simulink model "untitled"  (R2021a)
settings: Solver=VariableStepAuto  StartTime=0.0  StopTime=10.0  RelTol=1e-3
settings Model: Creator=ThinkPad  LastModifiedBy=ThinkPad

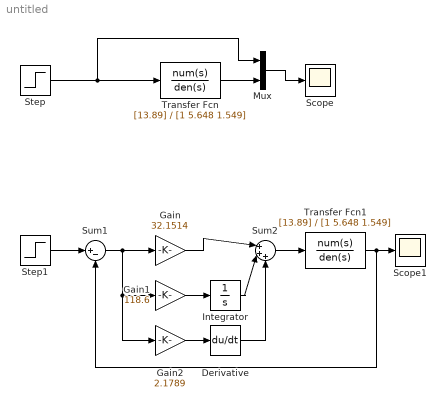
== system untitled ==
  Derivative : Derivative
  Gain : Gain  Gain=32.1514
  Gain1 : Gain  Gain=118.6
  Gain2 : Gain  Gain=2.1789
  Integrator : Integrator
  Mux : Mux  Inputs=2
  Scope : Scope
  Scope1 : Scope
  Step : Step  SampleTime=0
  Step1 : Step  SampleTime=0
  Sum1 : Sum  Inputs=|+-
  Sum2 : Sum  Inputs=|+++
  Transfer Fcn : TransferFcn  Numerator=[13.89]  Denominator=[1 5.648 1.549]
  Transfer Fcn1 : TransferFcn  Numerator=[13.89]  Denominator=[1 5.648 1.549]
  wires:
  Step/1 -> Mux/1, Transfer Fcn/1
  Step1/1 -> Sum1/1
  Sum1/1 -> Gain2/1, Gain1/1, Gain/1
  Sum2/1 -> Transfer Fcn1/1
  Gain/1 -> Sum2/1
  Gain1/1 -> Integrator/1
  Integrator/1 -> Sum2/2
  Gain2/1 -> Derivative/1
  Derivative/1 -> Sum2/3
  Transfer Fcn1/1 -> Sum1/2, Scope1/1
  Mux/1 -> Scope/1
  Transfer Fcn/1 -> Mux/2
